simulink model "model_sysid_admittance"  (R2016b)
settings: Solver=FixedStepDiscrete  StartTime=0.0  StopTime=inf  FixedStep=sampleTime  RelTol=1e-3
PostLoadFcn:
  | % load model parameters
  | % pname = fileparts(get_param('model_base_bros','filename'));
  | % run([pname  '\parameters_base_model_bros.m']);
  | parameters_sysid_admittance;
  | 
  | % set requested state
  | set_param('model_sysid_admittance/Requested state','Value',num2str(0));
InitFcn:
  | % load model parameters
  | % pname = fileparts(get_param('model_base_bros','filename'));
  | % run([pname  '\parameters_base_model_bros.m']);
  | parameters_sysid_admittance;
  | 
  | % set requested state
  | set_param('model_sysid_admittance/Requested state','Value',num2str(0));
StartFcn:
  | parameters_sysid_admittance;
  | 
  | % set requested state
  | set_param('model_sysid_admittance/Requested state','Value',num2str(0));
values from neighbouring files (symbols this model uses):
  Ax = [0.00153392997769 0.00153392997769 0.00153392997769 0.00153392997769 0.00153392997769 0.00153392997769 0.00153392997769 0.00153392997769 0.00153392997769 0.00153392997769 0.00153392997769 0.00153392997769 ... (25 elements, 25x1)]    [data_inputsignal_admittance_100Hz.mat]
  Ay = [0.00153392997769 0.00153392997769 0.00153392997769 0.00153392997769 0.00153392997769 0.00153392997769 0.00153392997769 0.00153392997769 0.00153392997769 0.00153392997769 0.00153392997769 0.00153392997769 ... (25 elements, 25x1)]    [data_inputsignal_admittance_100Hz.mat]
  Lb = 0.07    [model_affc_parameters.m]    (also in parameters_sysid.m; parameters_sysid_admittance.m)
  Lf = 0.238    [model_affc_parameters.m]    (also in parameters_sysid.m; parameters_sysid_admittance.m)
  Lu = 0.153    [model_affc_parameters.m]    (also in parameters_sysid.m; parameters_sysid_admittance.m)
  nx = [5 7 11 13 17 23 29 37 47 61 79 103 ... (25 elements, 25x1)]    [data_inputsignal_admittance_100Hz.mat]
  ny = [3 8 10 14 19 24 31 41 53 67 83 107 ... (25 elements, 25x1)]    [data_inputsignal_admittance_100Hz.mat]
  phx = [1.20009664335 1.06282811403 1.3892882876 -0.190948998613 4.36135308948 3.55125265665 -1.29943418487 -0.0100316069113 1.01892216761 0.472716168264 1.16765179672 3.48382334533 ... (25 elements, 25x1)]    [data_inputsignal_admittance_100Hz.mat]
  phy = [4.61290873425 3.09865303555 -1.33576318949 -0.454866147562 0.315570179572 -1.54269258334 1.9231806523 3.28701306913 -0.551495079422 2.37779557242 1.0737629469 -1.42157877686 ... (25 elements, 25x1)]    [data_inputsignal_admittance_100Hz.mat]
  sampleTime = 0.001    [model_affc_parameters.m]    (also in parameters_sysid.m; parameters_sysid_admittance.m)
  Tm = 12    [data_inputsignal.mat]    (also in data_inputsignal_100Hz.mat; data_inputsignal_100Hz_n40.mat; data_inputsignal_150Hz_n50.mat; data_inputsignal_50Hz.mat)
undefined symbols (not defined in the file or in its folder): BROS3
libraries: simulink x14, LibraryFM x7, VariousBlocksLibrary x6, simulink_extras x1
(part 1 of 2)
settings Model: SimulationMode=external  Creator=niekbeckers  LastModifiedBy=Labuser
settings DataIOCC: LimitDataPoints=on  SaveFormat=Array
settings OptimizationCC: BlockReduction=off  BooleanDataType=off  LocalBlockOutputs=off  LifeSpan=inf
settings DebuggingCC: SaveWithParameterizedLinksMsg=none  UnderspecifiedInitializationDetection=Classic  MergeDetectMultiDrivingBlocksExec=none  SignalResolutionControl=TryResolveAllWithWarning  SFUnexpectedBacktrackingDiag=warning  SFNoUnconditionalDefaultTransitionDiag=warning  SFExecutionAtInitializationDiag=none
settings HardwareCC: ProdBitPerPointer=32  ProdBitPerSizeT=32  ProdBitPerPtrDiffT=32  ProdLargestAtomicFloat=None  ProdIntDivRoundTo=Undefined  ProdEndianess=Unspecified  ProdWordSize=32  ProdHWDeviceType=32-bit Generic  TargetBitPerPointer=64  TargetBitPerSizeT=64  TargetBitPerPtrDiffT=64  TargetLongLongMode=on  TargetIntDivRoundTo=Zero  TargetEndianess=LittleEndian  TargetWordSize=64  TargetHWDeviceType=MATLAB Host  ProdEqTarget=off
settings ModelReferenceCC: PropagateSignalLabelsOutOfModel=off
settings RTWCC: SystemTargetFile=TwinCAT.tlc  GenCodeOnly=on  MakeCommand=make_tct  TemplateMakefile=tct_msbuild.tmf  Description=TwinCAT Target  GenerateReport=on  TargetLang=C++
settings STFCustomTargetCC: CompOptLevelCompliant=on  GeneratePreprocessorConditionals=Disable all  MATLABClassNameForMDSCustomization=Simulink.SoftwareTarget.TargetSpecificTriggerConfigurationBase  SystemTargetFile=TwinCAT.tlc
settings ConfigComp: CovMetricSettings=dw  CovHtmlReporting=on  CovSaveCumulativeToWorkspaceVar=on  CovSaveSingleToWorkspaceVar=on  CovExternalEMLEnable=off  CovSFcnEnable=off

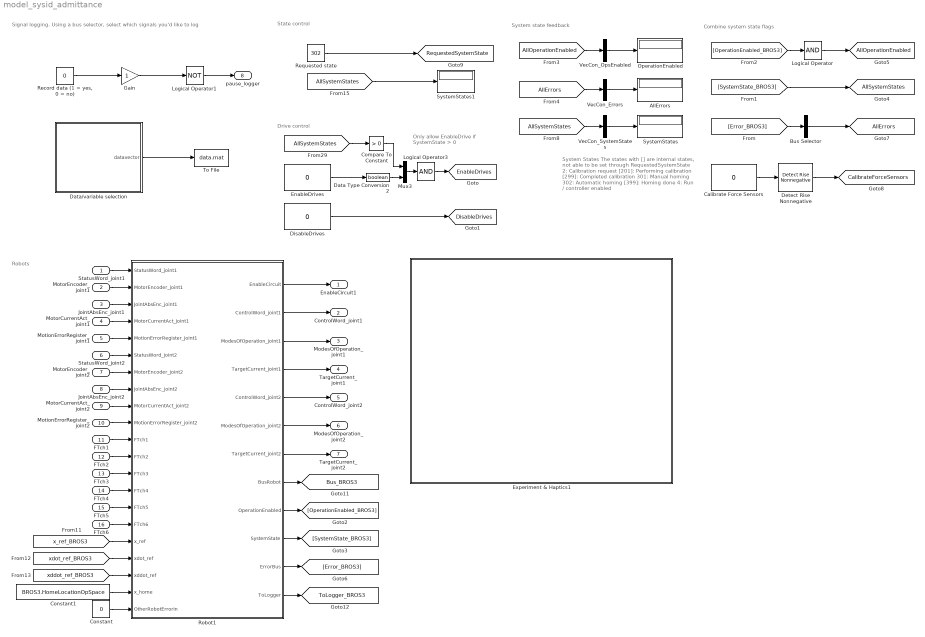
== system model_sysid_admittance ==
  note: Drive control
  note: System state feedback
  note: Only allow EnableDrive
      | if SystemState > 0
  note: Signal logging.
      | Using a bus selector, select which signals you'd like to log
  note: System States
      | The states with [] are internal states, not able to be set through RequestedSystemState
      | 2: Calibration request
      | [201]: Performing calibration
      | [299]: Completed calibration
      | 301: Manual homing
      | 302: Automatic homing
      | [399]: Homing done
      | 4: Run / controller enabled
  note: State control
  note: Combine system state flags
  note: Robots
  StatusWord_joint1 : Inport  OutDataTypeStr=uint16  PortDimensions=1
  MotorEncoder_joint1 : Inport  Port=2  OutDataTypeStr=int32  PortDimensions=1
  JointAbsEnc_joint1 : Inport  Port=3  OutDataTypeStr=int32  PortDimensions=1
  MotorCurrentAct_joint1 : Inport  Port=4  OutDataTypeStr=int16  PortDimensions=1
  MotionErrorRegister_joint1 : Inport  Port=5  OutDataTypeStr=uint16  PortDimensions=1
  StatusWord_joint2 : Inport  Port=6  OutDataTypeStr=uint16  PortDimensions=1
  MotorEncoder_joint2 : Inport  Port=7  OutDataTypeStr=int32  PortDimensions=1
  JointAbsEnc_joint2 : Inport  Port=8  OutDataTypeStr=int32  PortDimensions=1
  MotorCurrentAct_joint2 : Inport  Port=9  OutDataTypeStr=int16  PortDimensions=1
  MotionErrorRegister_joint2 : Inport  Port=10  OutDataTypeStr=uint16  PortDimensions=1
  FTch1 : Inport  Port=11  OutDataTypeStr=single  PortDimensions=1
  FTch2 : Inport  Port=12  OutDataTypeStr=single  PortDimensions=1
  FTch3 : Inport  Port=13  OutDataTypeStr=single  PortDimensions=1
  FTch4 : Inport  Port=14  OutDataTypeStr=single  PortDimensions=1
  FTch5 : Inport  Port=15  OutDataTypeStr=single  PortDimensions=1
  FTch6 : Inport  Port=16  OutDataTypeStr=single  PortDimensions=1
  AllErrors : Display
  Bus Selector : BusSelector  OutputSignals=ErrorCodeLatched  OutputAsBus=on
  Calibrate Force Sensors : Constant  Value=0
      settings: OpenFcn=set_param(gcb,'Value','1');tname = ['toggletimer_' gcb];delete(timerfind('name',tname));t = timer('timerfcn', ['set_param(''',gcb,''',''Value'',''0'')'],'executionmode','singleshot','startdelay',1,'name',tname);start(t);
      mask Display: fprintf('PushToTrigger\n%s',get_param(gcb,'value'))
  Compare To Constant : simulink/Logic and Bit Operations/Compare To Constant  relop=>  const=0  OutDataTypeStr=boolean
  Constant : Constant  Value=0
  Constant1 : Constant  Value=BROS3.HomeLocationOpSpace
  Data Type Conversion2 : DataTypeConversion  OutDataTypeStr=boolean
  Data/variable selection : Subsystem
  Detect Rise Nonnegative : simulink/Logic and Bit Operations/Detect Rise Nonnegative  vinit=0  OutDataTypeStr=boolean
  DisableDrives : Constant  Value=0
      settings: OpenFcn=set_param(gcb,'Value','1');tname = ['toggletimer_' gcb];delete(timerfind('name',tname));t = timer('timerfcn', ['set_param(''',gcb,''',''Value'',''0'')'],'executionmode','singleshot','startdelay',1,'name',tname);start(t);
      mask Display: fprintf('PushToTrigger\n%s',get_param(gcb,'value'))
  EnableDrives : Constant  Value=0
      settings: OpenFcn=set_param(gcb,'Value','1');tname = ['toggletimer_' gcb];delete(timerfind('name',tname));t = timer('timerfcn', ['set_param(''',gcb,''',''Value'',''0'')'],'executionmode','singleshot','startdelay',1,'name',tname);start(t);
      mask Display: fprintf('PushToTrigger\n%s',get_param(gcb,'value'))
  Experiment & Haptics1 : Subsystem
  Gain : Gain
  Logical Operator : Logic  Inputs=1  AllPortsSameDT=off  OutDataTypeStr=boolean
  Logical Operator1 : Logic  Operator=NOT  Inputs=1  AllPortsSameDT=off  OutDataTypeStr=boolean
  Logical Operator3 : Logic  Inputs=1  AllPortsSameDT=off  OutDataTypeStr=boolean
  Mux3 : Mux  Inputs=2
  OperationEnabled : Display
  "Record data (1 = yes, 0 = no)" : Constant  Value=0  OutDataTypeStr=boolean
  Requested state : Constant  Value=302
  Robot1 : Subsystem  mask{RobotStruct=BROS3}
      mask prompts: RobotStruct "Robot struct (data)"
  SystemStates : Display
  SystemStates1 : Display
  To File : ToFile  Filename=data.mat  MatrixName=data
  VecCon_Errors : Concatenate  NumInputs=1
  VecCon_OpsEnabled : Concatenate  NumInputs=1
  VecCon_SystemStates : Concatenate  NumInputs=1
  EnableCircuit1 : Outport  OutDataTypeStr=boolean  PortDimensions=1
  ControlWord_joint1 : Outport  Port=2  OutDataTypeStr=uint16  PortDimensions=1
  ModesOfOperation_joint1 : Outport  Port=3  OutDataTypeStr=int8  PortDimensions=1
  TargetCurrent_joint1 : Outport  Port=4  OutDataTypeStr=int16  PortDimensions=1
  ControlWord_joint2 : Outport  Port=5  OutDataTypeStr=uint16  PortDimensions=1
  ModesOfOperation_joint2 : Outport  Port=6  OutDataTypeStr=int8  PortDimensions=1
  TargetCurrent_joint2 : Outport  Port=7  OutDataTypeStr=int16  PortDimensions=1
  pause_logger : Outport  Port=8  OutDataTypeStr=boolean  PortDimensions=1
  tag scope: AllErrors=global, AllOperationEnabled=global, AllSystemStates=global, Bus_BROS3=global, CalibrateForceSensors=global, DisableDrives=global, EnableDrives=global, RequestedSystemState=global, ToLogger_BROS3=global
  wires:
  DisableDrives/1 -> [DisableDrives]
  Robot1/9(OperationEnabled) -> [OperationEnabled_BROS3]
  [AllOperationEnabled] -> VecCon_OpsEnabled/1
  Robot1/10(SystemState) -> [SystemState_BROS3]
  [SystemState_BROS3] -> [AllSystemStates]
  Logical Operator/1 -> [AllOperationEnabled]
  [OperationEnabled_BROS3] -> Logical Operator/1
  [Error_BROS3] -> Bus Selector/1
  [AllErrors] -> VecCon_Errors/1
  [x_ref_BROS3] -> Robot1/17(x_ref)
  [xdot_ref_BROS3] -> Robot1/18(xdot_ref)
  [xddot_ref_BROS3] -> Robot1/19(xddot_ref)
  Requested state/1 -> [RequestedSystemState]
  Robot1/8(BusRobot) -> [Bus_BROS3]
  StatusWord_joint1/1 -> Robot1/1(StatusWord_joint1)
  MotorEncoder_joint1/1 -> Robot1/2(MotorEncoder_joint1)
  JointAbsEnc_joint1/1 -> Robot1/3(JointAbsEnc_joint1)
  MotorCurrentAct_joint1/1 -> Robot1/4(MotorCurrentAct_joint1)
  StatusWord_joint2/1 -> Robot1/6(StatusWord_joint2)
  MotorEncoder_joint2/1 -> Robot1/7(MotorEncoder_joint2)
  JointAbsEnc_joint2/1 -> Robot1/8(JointAbsEnc_joint2)
  MotorCurrentAct_joint2/1 -> Robot1/9(MotorCurrentAct_joint2)
  FTch1/1 -> Robot1/11(FTch1)
  FTch2/1 -> Robot1/12(FTch2)
  FTch3/1 -> Robot1/13(FTch3)
  FTch4/1 -> Robot1/14(FTch4)
  FTch5/1 -> Robot1/15(FTch5)
  FTch6/1 -> Robot1/16(FTch6)
  Robot1/2(ControlWord_joint1) -> ControlWord_joint1/1
  Robot1/3(ModesOfOperation_joint1) -> ModesOfOperation_joint1/1
  Robot1/4(TargetCurrent_joint1) -> TargetCurrent_joint1/1
  Robot1/7(TargetCurrent_joint2) -> TargetCurrent_joint2/1
  Robot1/6(ModesOfOperation_joint2) -> ModesOfOperation_joint2/1
  Robot1/5(ControlWord_joint2) -> ControlWord_joint2/1
  [AllSystemStates] -> SystemStates1/1
  Logical Operator1/1 -> pause_logger/1
  Bus Selector/1 -> [AllErrors]
  Robot1/1(EnableCircuit) -> EnableCircuit1/1
  VecCon_Errors/1 -> AllErrors/1
  [AllSystemStates] -> VecCon_SystemStates/1
  VecCon_SystemStates/1 -> SystemStates/1
  VecCon_OpsEnabled/1 -> OperationEnabled/1
  [AllSystemStates] -> Compare To Constant/1
  Logical Operator3/1 -> [EnableDrives]
  EnableDrives/1 -> Data Type Conversion2/1
  Compare To Constant/1 -> Mux3/1
  Mux3/1 -> Logical Operator3/1
  Data Type Conversion2/1 -> Mux3/2
  Constant1/1 -> Robot1/20(x_home)
  Data/variable selection/1(datavector) -> To File/1
  Constant/1 -> Robot1/21(OtherRobotErrorIn)
  Calibrate Force Sensors/1 -> Detect Rise Nonnegative/1
  Detect Rise Nonnegative/1 -> [CalibrateForceSensors]
  Robot1/12(ToLogger) -> [ToLogger_BROS3]
  Robot1/11(ErrorBus) -> [Error_BROS3]
  MotionErrorRegister_joint1/1 -> Robot1/5(MotionErrorRegister_joint1)
  MotionErrorRegister_joint2/1 -> Robot1/10(MotionErrorRegister_joint2)
  "Record data (1 = yes, 0 = no)"/1 -> Gain/1
  Gain/1 -> Logical Operator1/1

== system model_sysid_admittance/Data//variable selection ==
  Bus to Vector : BusToVector
  BusSelectorLoggerBROS1 : BusSelector  OutputSignals=SystemState,qJointSpace.q_AbsEnc,qJointSpace.qdot_AbsEnc,qJointSpace.q_IncEnc,qJointSpace.qdot_IncEnc,xOpSpace.x_AbsEnc,xOpSpace.xdot_AbsEnc,xOpSpace.x,xOpSpace.xdot,Controller_ToLogger.x_ref,Controller_ToLogger.xdot_ref,Controller_ToLogger.xddot_ref,qJointSpace.JointTorque_Nm,BusFTSensor.ForcesOpSpace  OutputAsBus=on
  Mux5 : Mux  Inputs=3
  datavector : Outport
  wires:
  BusSelectorLoggerBROS1/1 -> Bus to Vector/1
  [ToLogger_BROS3] -> BusSelectorLoggerBROS1/1
  [AllErrors] -> Mux5/2
  Bus to Vector/1 -> Mux5/1
  Mux5/1 -> datavector/1
  [ExpData] -> Mux5/3

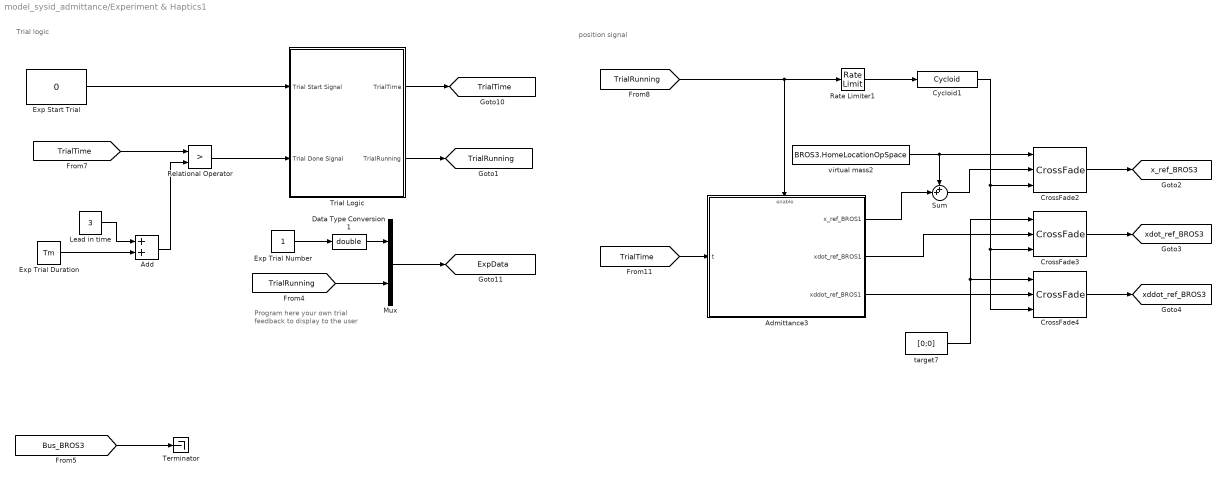
== system model_sysid_admittance/Experiment & Haptics1 ==
  note: Program here your own trial
      | feedback to display to the user
  note: Trial logic
  note: position signal
  Add : Sum
  Admittance3 : Subsystem
  CrossFade2 : VariousBlocksLibrary/Various/CrossFade
  CrossFade3 : VariousBlocksLibrary/Various/CrossFade
  CrossFade4 : VariousBlocksLibrary/Various/CrossFade
  Cycloid1 : VariousBlocksLibrary/Various/Cycloid
  Data Type Conversion1 : DataTypeConversion  OutDataTypeStr=double
  Exp Start Trial : Constant  Value=0
      settings: OpenFcn=set_param(gcb,'Value','1');tname = ['toggletimer_' gcb];delete(timerfind('name',tname));t = timer('timerfcn', ['set_param(''',gcb,''',''Value'',''0'')'],'executionmode','singleshot','startdelay',1,'name',tname);start(t);
      mask Display: fprintf('PushToTrigger\n%s',get_param(gcb,'value'))
  Exp Trial Duration : Constant  Value=Tm  OutDataTypeStr=double
  Exp Trial Number : Constant  OutDataTypeStr=int32
  Lead in time : Constant  Value=3  OutDataTypeStr=double
  Mux : Mux  Inputs=2
  Rate Limiter1 : RateLimiter  RisingSlewLimit=1/3.0  FallingSlewLimit=-1/3.0  SampleTimeMode=inherited
  Relational Operator : RelationalOperator  Operator=>  OutDataTypeStr=boolean  RndMeth=Simplest
  Sum : Sum  Inputs=++|
  Terminator : Terminator
  Trial Logic : Subsystem
  target7 : Constant  Value=[0;0]
  virtual mass2 : Constant  Value=BROS3.HomeLocationOpSpace
  tag scope: ExpData=global, TrialRunning=global, TrialTime=global, x_ref_BROS3=global, xddot_ref_BROS3=global, xdot_ref_BROS3=global
  wires:
  Mux/1 -> [ExpData]
  Exp Trial Number/1 -> Data Type Conversion1/1
  [TrialRunning] -> Mux/2
  Data Type Conversion1/1 -> Mux/1
  Exp Trial Duration/1 -> Add/2
  Exp Start Trial/1 -> Trial Logic/1(Trial Start Signal)
  Trial Logic/1(TrialTime) -> [TrialTime]
  Trial Logic/2(TrialRunning) -> [TrialRunning]
  Relational Operator/1 -> Trial Logic/2(Trial Done Signal)
  CrossFade2/1 -> [x_ref_BROS3]
  CrossFade3/1 -> [xdot_ref_BROS3]
  CrossFade4/1 -> [xddot_ref_BROS3]
  Add/1 -> Relational Operator/2
  Lead in time/1 -> Add/1
  [TrialTime] -> Relational Operator/1
  [TrialRunning] -> Rate Limiter1/1, Admittance3/Enable
  Cycloid1/1 -> CrossFade3/3, CrossFade4/3, CrossFade2/3
  Rate Limiter1/1 -> Cycloid1/1
  virtual mass2/1 -> CrossFade2/1, Sum/1
  target7/1 -> CrossFade3/1, CrossFade4/1
  Admittance3/2(xdot_ref_BROS1) -> CrossFade3/2
  Admittance3/3(xddot_ref_BROS1) -> CrossFade4/2
  [TrialTime] -> Admittance3/1(t)
  Admittance3/1(x_ref_BROS1) -> Sum/2
  Sum/1 -> CrossFade2/2
  [Bus_BROS3] -> Terminator/1

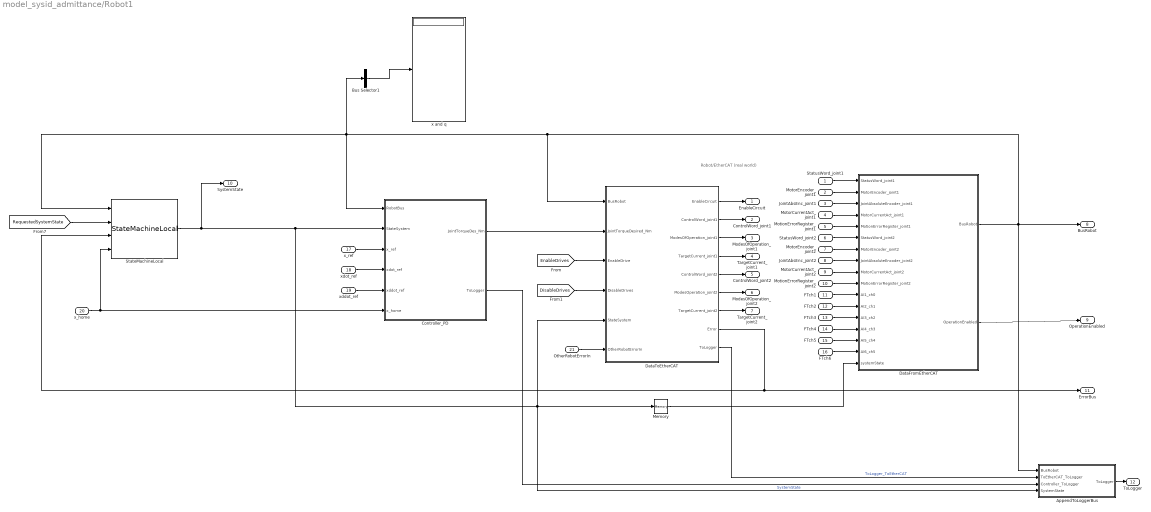
== system model_sysid_admittance/Robot1 ==
  note: Robot/EtherCAT (real world)
  StatusWord_joint1 : Inport
  MotorEncoder_joint1 : Inport  Port=2
  JointAbsEnc_joint1 : Inport  Port=3
  MotorCurrentAct_joint1 : Inport  Port=4
  MotionErrorRegister_joint1 : Inport  Port=5  OutDataTypeStr=uint16
  StatusWord_joint2 : Inport  Port=6
  MotorEncoder_joint2 : Inport  Port=7
  JointAbsEnc_joint2 : Inport  Port=8
  MotorCurrentAct_joint2 : Inport  Port=9
  MotionErrorRegister_joint2 : Inport  Port=10  OutDataTypeStr=uint16
  FTch1 : Inport  Port=11
  FTch2 : Inport  Port=12
  FTch3 : Inport  Port=13
  FTch4 : Inport  Port=14
  FTch5 : Inport  Port=15
  FTch6 : Inport  Port=16
  x_ref : Inport  Port=17
  xdot_ref : Inport  Port=18
  xddot_ref : Inport  Port=19
  x_home : Inport  Port=20
  OtherRobotErrorIn : Inport  Port=21
  AppendToLoggerBus : Subsystem
  Bus Selector1 : BusSelector  OutputSignals=qJointSpace.q_AbsEnc,qJointSpace.qdot_AbsEnc,xOpSpace.x,BusActuators.BusActuator1.JointPosition_AbsEnc_rad,BusActuators.BusActuator2.JointPosition_AbsEnc_rad,qJointSpace.q_IncEnc,qJointSpace.qdot_IncEnc  OutputAsBus=on
  Controller_PD : Subsystem
  DataFromEtherCAT : Subsystem
  DataToEtherCAT : Subsystem
  Memory : Memory
  StateMachineLocal : LibraryFM/StateMachineLocal
  x and q : Display
  EnableCircuit : Outport
  ControlWord_joint1 : Outport  Port=2
  ModesOfOperation_joint1 : Outport  Port=3
  TargetCurrent_joint1 : Outport  Port=4
  ControlWord_joint2 : Outport  Port=5
  ModesOfOperation_joint2 : Outport  Port=6
  TargetCurrent_joint2 : Outport  Port=7
  BusRobot : Outport  Port=8
  OperationEnabled : Outport  Port=9
  SystemState : Outport  Port=10
  ErrorBus : Outport  Port=11
  ToLogger : Outport  Port=12
  wires:
  xddot_ref/1 -> Controller_PD/5(xddot_ref)
  xdot_ref/1 -> Controller_PD/4(xdot_ref)
  x_ref/1 -> Controller_PD/3(x_ref)
  DataToEtherCAT/7(TargetCurrent_joint2) -> TargetCurrent_joint2/1
  FTch2/1 -> DataFromEtherCAT/12(AI2_ch1)
  MotorCurrentAct_joint1/1 -> DataFromEtherCAT/4(MotorCurrentAct_joint1)
  MotorEncoder_joint2/1 -> DataFromEtherCAT/7(MotorEncoder_joint2)
  JointAbsEnc_joint1/1 -> DataFromEtherCAT/3(JointAbsoluteEncoder_joint1)
  DataToEtherCAT/3(ModesOfOperation_joint1) -> ModesOfOperation_joint1/1
  DataToEtherCAT/1(EnableCircuit) -> EnableCircuit/1
  FTch1/1 -> DataFromEtherCAT/11(AI1_ch0)
  StateMachineLocal/1 -> Controller_PD/2(StateSystem), DataToEtherCAT/5(StateSystem), Memory/1, AppendToLoggerBus/4(SystemState), SystemState/1  "SystemState"
  DataToEtherCAT/2(ControlWord_joint1) -> ControlWord_joint1/1
  DataToEtherCAT/8(Error) -> StateMachineLocal/3, ErrorBus/1
  DataFromEtherCAT/1(BusRobot) -> AppendToLoggerBus/1(BusRobot), Controller_PD/1(RobotBus), Bus Selector1/1, StateMachineLocal/1, DataToEtherCAT/1(BusRobot), BusRobot/1
  [RequestedSystemState] -> StateMachineLocal/2
  Controller_PD/1(JointTorqueDes_Nm) -> DataToEtherCAT/2(JointTorqueDesired_Nm)
  [DisableDrives] -> DataToEtherCAT/4(DisableDrives)
  [EnableDrives] -> DataToEtherCAT/3(EnableDrive)
  MotorCurrentAct_joint2/1 -> DataFromEtherCAT/9(MotorCurrentAct_joint2)
  DataToEtherCAT/4(TargetCurrent_joint1) -> TargetCurrent_joint1/1
  FTch5/1 -> DataFromEtherCAT/15(AI5_ch4)
  JointAbsEnc_joint2/1 -> DataFromEtherCAT/8("JointAbsoluteEncoder_joint2 ")
  MotorEncoder_joint1/1 -> DataFromEtherCAT/2(MotorEncoder_joint1)
  DataToEtherCAT/5(ControlWord_joint2) -> ControlWord_joint2/1
  DataToEtherCAT/6(ModesOperation_joint2) -> ModesOfOperation_joint2/1
  StatusWord_joint1/1 -> DataFromEtherCAT/1(StatusWord_joint1)
  StatusWord_joint2/1 -> DataFromEtherCAT/6(StatusWord_joint2)
  FTch6/1 -> DataFromEtherCAT/16(AI6_ch5)
  FTch4/1 -> DataFromEtherCAT/14(AI4_ch3)
  FTch3/1 -> DataFromEtherCAT/13(AI3_ch2)
  DataFromEtherCAT/2(OperationEnabled) -> OperationEnabled/1
  Bus Selector1/1 -> x and q/1
  Controller_PD/2(ToLogger) -> AppendToLoggerBus/3(Controller_ToLogger)
  DataToEtherCAT/9(ToLogger) -> AppendToLoggerBus/2(ToEtherCAT_ToLogger)  "ToLogger_ToEtherCAT"
  AppendToLoggerBus/1(ToLogger) -> ToLogger/1
  Memory/1 -> DataFromEtherCAT/17(systemState)
  OtherRobotErrorIn/1 -> DataToEtherCAT/6(OtherRobotErrorIn)
  x_home/1 -> StateMachineLocal/4, Controller_PD/6(x_home)
  MotionErrorRegister_joint1/1 -> DataFromEtherCAT/5(MotionErrorRegister_joint1)
  MotionErrorRegister_joint2/1 -> DataFromEtherCAT/10(MotionErrorRegister_joint2)

== system model_sysid_admittance/Experiment & Haptics1/Admittance3 ==
  t : Inport
  Enable : EnablePort  StatesWhenEnabling=reset
  Constant3 : Constant  Value=0.5
  MATLAB Function : MATLAB Function  TreatAsAtomicUnit=on
  Product : Product
  Product1 : Product
  Product2 : Product
  x_ref_BROS1 : Outport
  xdot_ref_BROS1 : Outport  Port=2
  xddot_ref_BROS1 : Outport  Port=3
  wires:
  Product/1 -> x_ref_BROS1/1
  MATLAB Function/1(p) -> Product/2
  t/1 -> MATLAB Function/1(t)
  Product1/1 -> xdot_ref_BROS1/1
  Product2/1 -> xddot_ref_BROS1/1
  MATLAB Function/2(v) -> Product1/2
  MATLAB Function/3(a) -> Product2/2
  Constant3/1 -> Product2/1, Product1/1, Product/1

== system model_sysid_admittance/Experiment & Haptics1/Trial Logic ==
  Trial Start Signal : Inport
  Trial Done Signal : Inport  Port=2
  CheckTrialIsRunning : simulink_extras/Flip Flops/S-R Flip-Flop  initial_condition=0
  Data Type Conversion : DataTypeConversion  OutDataTypeStr=double
  Detect Rise Positive : simulink/Logic and Bit Operations/Detect Rise Positive  vinit=0  OutDataTypeStr=boolean
  Detect Rise Positive1 : simulink/Logic and Bit Operations/Detect Rise Positive  vinit=0  OutDataTypeStr=boolean
  Logical Operator : Logic  AllPortsSameDT=off  OutDataTypeStr=boolean
  Memory : Memory
  StopWatch : Subsystem
  Terminator4 : Terminator
  TrialTime : Outport
  TrialRunning : Outport  Port=2
  wires:
  CheckTrialIsRunning/1 -> Memory/1, Data Type Conversion/1
  Memory/1 -> StopWatch/Enable, Logical Operator/1
  Trial Start Signal/1 -> Detect Rise Positive/1
  Detect Rise Positive1/1 -> CheckTrialIsRunning/2
  Detect Rise Positive/1 -> CheckTrialIsRunning/1
  StopWatch/1(trialTime) -> TrialTime/1
  CheckTrialIsRunning/2 -> Terminator4/1
  Data Type Conversion/1 -> TrialRunning/1
  Trial Done Signal/1 -> Logical Operator/2
  Logical Operator/1 -> Detect Rise Positive1/1

== system model_sysid_admittance/Robot1/AppendToLoggerBus ==
  BusRobot : Inport
  ToEtherCAT_ToLogger : Inport  Port=2
  Controller_ToLogger : Inport  Port=3
  SystemState : Inport  Port=4
  Bus Creator : BusCreator  Inputs=8
  Bus Selector : BusSelector  OutputSignals=xOpSpace,qJointSpace,BusFTSensor,BusActuators
  Bus Selector1 : BusSelector  OutputSignals=ToEtherCAT_ToLogger_Actuator1,ToEtherCAT_ToLogger_Actuator2
  ToLogger : Outport
  wires:
  Bus Creator/1 -> ToLogger/1  "LoggerBus"
  Bus Selector/4 -> Bus Creator/4  "<BusActuators>"
  Bus Selector/1 -> Bus Creator/1  "<xOpSpace>"
  Bus Selector/3 -> Bus Creator/3  "<BusFTSensor>"
  Bus Selector/2 -> Bus Creator/2  "<qJointSpace>"
  BusRobot/1 -> Bus Selector/1
  ToEtherCAT_ToLogger/1 -> Bus Selector1/1
  Bus Selector1/1 -> Bus Creator/5  "<ToEtherCAT_ToLogger_Actuator1>"
  Bus Selector1/2 -> Bus Creator/6  "<ToEtherCAT_ToLogger_Actuator2>"
  Controller_ToLogger/1 -> Bus Creator/7
  SystemState/1 -> Bus Creator/8  "SystemState"

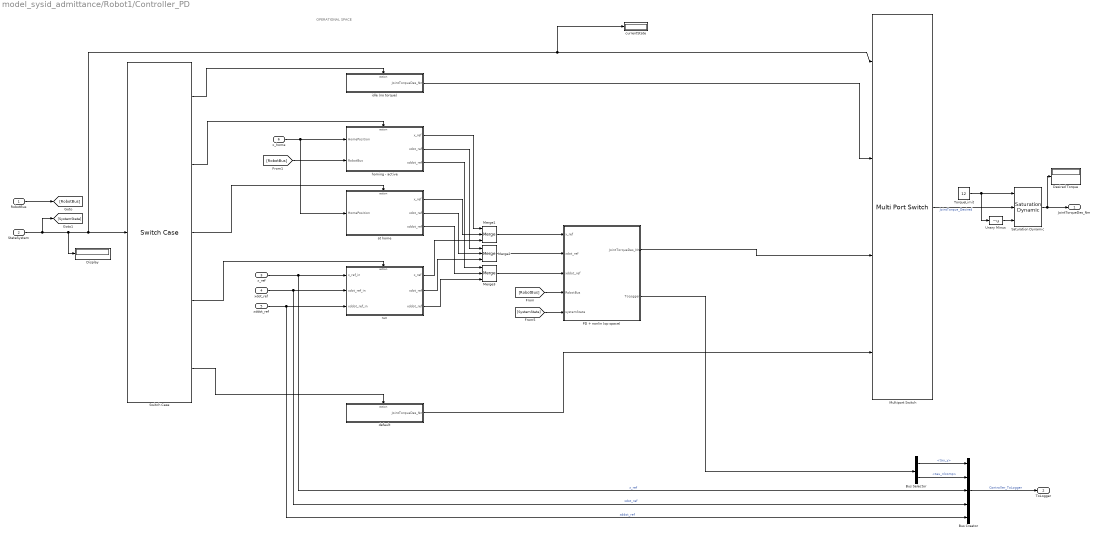
== system model_sysid_admittance/Robot1/Controller_PD ==
  note: OPERATIONAL SPACE
  RobotBus : Inport
  StateSystem : Inport  Port=2
  x_ref : Inport  Port=3
  xdot_ref : Inport  Port=4
  xddot_ref : Inport  Port=5
  x_home : Inport  Port=6
  Bus Creator : BusCreator  Inputs=5
  Bus Selector : BusSelector  OutputSignals=tau_y,tau_nlcomp
  Desired Torque : Display
  Display : Display
  Merge1 : Merge  Inputs=3  InitialOutput=[0;0]
  Merge2 : Merge  Inputs=3  InitialOutput=[0;0]
  Merge3 : Merge  Inputs=3  InitialOutput=[0;0]
  Multiport Switch : MultiPortSwitch  DataPortOrder=Specify indices  Inputs=4  DataPortIndices={[0,1,2,201,299,301],[302,399,4]}  DataPortForDefault=Additional data port
  PD + nonlin (op space) : Subsystem
  Saturation Dynamic : simulink/Discontinuities/Saturation Dynamic  OutMin=[]  OutMax=[]  OutDataTypeStr=Inherit: Same as second input  OutDataType=fixdt(1, 16)  OutScaling=2^-10  DoSatur=off
  Switch Case : SwitchCase  CaseConditions={[0,1,2,201,299,301],302, 399,[4]}
  TorqueLimit : Constant  Value=12
  Unary Minus : UnaryMinus
  at home : Subsystem
  currentState : Display
  default : Subsystem  TreatAsAtomicUnit=on
  homing - active : Subsystem
  idle (no torque) : Subsystem  TreatAsAtomicUnit=on
  run : Subsystem
  JointTorqueDes_Nm : Outport
  ToLogger : Outport  Port=2
  wires:
  [SystemState] -> PD + nonlin (op space)/5(systemState)
  xddot_ref/1 -> Bus Creator/5, run/3(xddot_ref_in)  "xddot_ref"
  xdot_ref/1 -> Bus Creator/4, run/2(xdot_ref_in)  "xdot_ref"
  x_ref/1 -> Bus Creator/3, run/1(x_ref_in)  "x_ref"
  [RobotBus] -> PD + nonlin (op space)/4(RobotBus)
  RobotBus/1 -> [RobotBus]
  Merge3/1 -> PD + nonlin (op space)/3(xddot_ref)
  Merge2/1 -> PD + nonlin (op space)/2(xdot_ref)
  Merge1/1 -> PD + nonlin (op space)/1(x_ref)
  idle (no torque)/1(JointTorqueDes_Nm) -> Multiport Switch/2
  Switch Case/2 -> homing - active/Action
  Switch Case/1 -> idle (no torque)/Action
  default/1(JointTorqueDes_Nm) -> Multiport Switch/4
  Switch Case/5 -> default/Action
  Saturation Dynamic/1 -> Desired Torque/1, JointTorqueDes_Nm/1
  Switch Case/3 -> at home/Action
  homing - active/1(x_ref) -> Merge1/1
  run/1(x_ref) -> Merge1/3
  StateSystem/1 -> Display/1, Multiport Switch/1, currentState/1, Switch Case/1, [SystemState]
  run/2(xdot_ref) -> Merge2/3
  run/3(xddot_ref) -> Merge3/3
  homing - active/2(xdot_ref) -> Merge2/1
  homing - active/3(xddot_ref) -> Merge3/1
  Multiport Switch/1 -> Saturation Dynamic/2  "JointTorque_Desired"
  PD + nonlin (op space)/2(ToLogger) -> Bus Selector/1
  x_home/1 -> at home/1(HomePosition), homing - active/1(HomePosition)
  Bus Creator/1 -> ToLogger/1  "Controller_ToLogger"
  Bus Selector/1 -> Bus Creator/1  "<tau_y>"
  Bus Selector/2 -> Bus Creator/2  "<tau_nlcomp>"
  TorqueLimit/1 -> Unary Minus/1, Saturation Dynamic/1
  Unary Minus/1 -> Saturation Dynamic/3
  [RobotBus] -> homing - active/2(RobotBus)
  at home/1(x_ref) -> Merge1/2
  at home/2(xdot_ref) -> Merge2/2
  at home/3(xddot_ref) -> Merge3/2
  Switch Case/4 -> run/Action
  PD + nonlin (op space)/1(JointTorqueDes_Nm) -> Multiport Switch/3

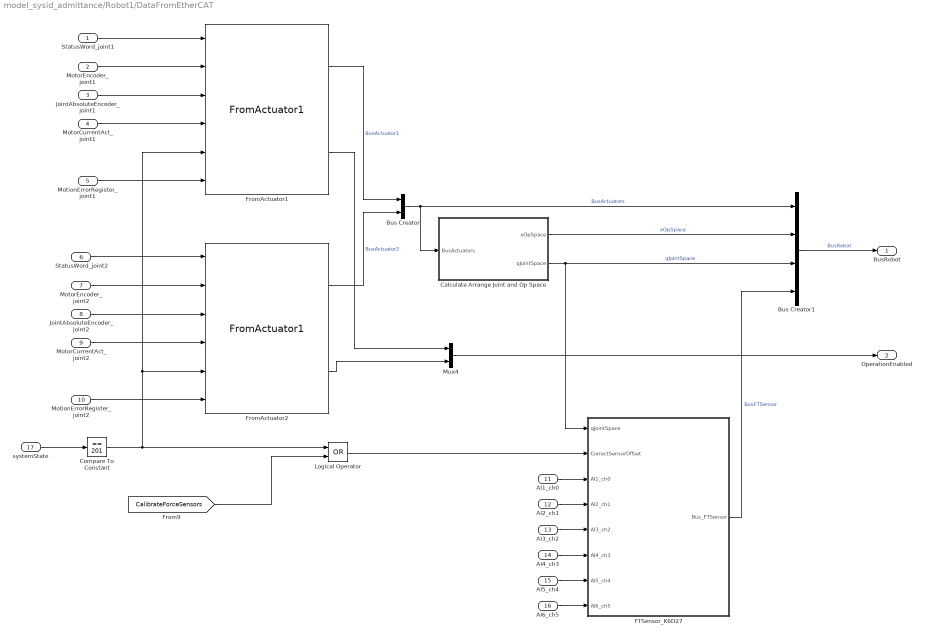
== system model_sysid_admittance/Robot1/DataFromEtherCAT ==
  StatusWord_joint1 : Inport
  MotorEncoder_joint1 : Inport  Port=2
  JointAbsoluteEncoder_joint1 : Inport  Port=3
  MotorCurrentAct_joint1 : Inport  Port=4
  MotionErrorRegister_joint1 : Inport  Port=5  OutDataTypeStr=uint16
  StatusWord_joint2 : Inport  Port=6
  MotorEncoder_joint2 : Inport  Port=7
  "JointAbsoluteEncoder_joint2 " : Inport  Port=8
  MotorCurrentAct_joint2 : Inport  Port=9
  MotionErrorRegister_joint2 : Inport  Port=10  OutDataTypeStr=uint16
  AI1_ch0 : Inport  Port=11
  AI2_ch1 : Inport  Port=12
  AI3_ch2 : Inport  Port=13
  AI4_ch3 : Inport  Port=14
  AI5_ch4 : Inport  Port=15
  AI6_ch5 : Inport  Port=16
  systemState : Inport  Port=17
  Bus Creator : BusCreator  Inputs=2
  Bus Creator1 : BusCreator  Inputs=4
  Calculate Arrange Joint and Op Space : Subsystem
  Compare To Constant : simulink/Logic and Bit Operations/Compare To Constant  relop===  const=201  OutDataTypeStr=boolean
  FTSensor_K6D27 : Subsystem  mask{FTSensorStruct=RobotStruct.FTSensor}
      mask prompts: FTSensorStruct "Struct for force torque sensor"
  FromActuator1 : LibraryFM/FromActuator1  ActuatorStruct=RobotStruct.Actuator1
  FromActuator2 : LibraryFM/FromActuator1  ActuatorStruct=RobotStruct.Actuator2
  Logical Operator : Logic  Operator=OR  AllPortsSameDT=off  OutDataTypeStr=boolean
  Mux4 : Mux  Inputs=2
  BusRobot : Outport
  OperationEnabled : Outport  Port=2
  wires:
  FTSensor_K6D27/1(Bus_FTSensor) -> Bus Creator1/4  "BusFTSensor"
  FromActuator1/1 -> Bus Creator/1  "BusActuator1"
  FromActuator2/1 -> Bus Creator/2  "BusActuator2"
  FromActuator1/2 -> Mux4/1
  Mux4/1 -> OperationEnabled/1
  FromActuator2/2 -> Mux4/2
  MotorEncoder_joint1/1 -> FromActuator1/2
  StatusWord_joint1/1 -> FromActuator1/1
  JointAbsoluteEncoder_joint1/1 -> FromActuator1/3
  MotorCurrentAct_joint1/1 -> FromActuator1/4
  MotorEncoder_joint2/1 -> FromActuator2/2
  StatusWord_joint2/1 -> FromActuator2/1
  "JointAbsoluteEncoder_joint2 "/1 -> FromActuator2/3
  MotorCurrentAct_joint2/1 -> FromActuator2/4
  Bus Creator/1 -> Calculate Arrange Joint and Op Space/1(BusActuators), Bus Creator1/1  "BusActuators"
  Bus Creator1/1 -> BusRobot/1  "BusRobot"
  Calculate Arrange Joint and Op Space/2(qJointSpace) -> FTSensor_K6D27/1(qJointSpace), Bus Creator1/3  "qJointSpace"
  systemState/1 -> Compare To Constant/1
  AI1_ch0/1 -> FTSensor_K6D27/3(AI1_ch0)
  AI2_ch1/1 -> FTSensor_K6D27/4(AI2_ch1)
  AI3_ch2/1 -> FTSensor_K6D27/5(AI3_ch2)
  AI4_ch3/1 -> FTSensor_K6D27/6(AI4_ch3)
  AI5_ch4/1 -> FTSensor_K6D27/7(AI5_ch4)
  AI6_ch5/1 -> FTSensor_K6D27/8(AI6_ch5)
  Compare To Constant/1 -> Logical Operator/1, FromActuator1/5, FromActuator2/5
  Calculate Arrange Joint and Op Space/1(xOpSpace) -> Bus Creator1/2  "xOpSpace"
  [CalibrateForceSensors] -> Logical Operator/2
  Logical Operator/1 -> FTSensor_K6D27/2(CorrectSensorOffset)
  MotionErrorRegister_joint1/1 -> FromActuator1/6
  MotionErrorRegister_joint2/1 -> FromActuator2/6

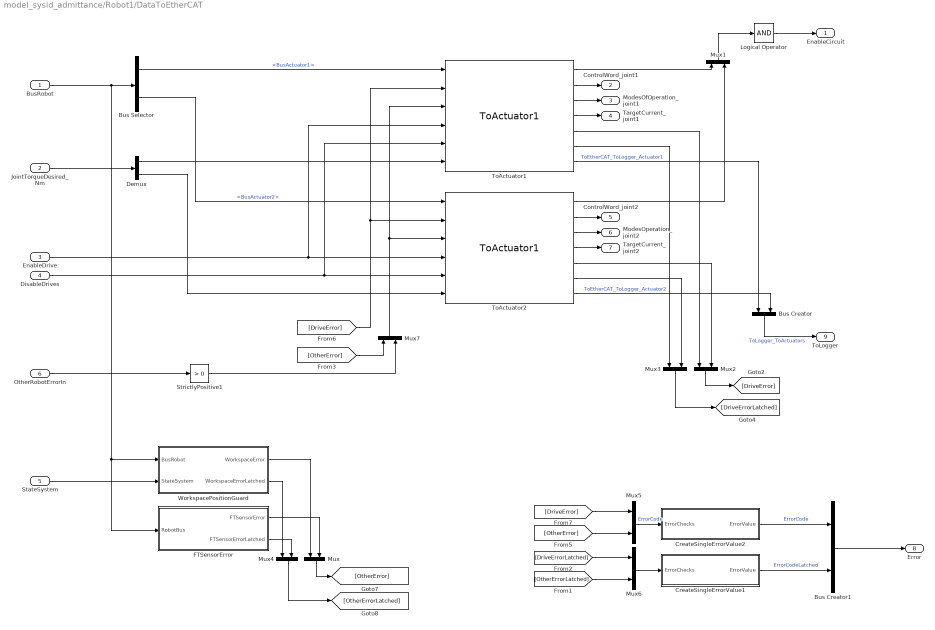
== system model_sysid_admittance/Robot1/DataToEtherCAT ==
  BusRobot : Inport
  JointTorqueDesired_Nm : Inport  Port=2
  EnableDrive : Inport  Port=3
  DisableDrives : Inport  Port=4
  StateSystem : Inport  Port=5
  OtherRobotErrorIn : Inport  Port=6
  Bus Creator : BusCreator  Inputs=2
  Bus Creator1 : BusCreator  Inputs=2
  Bus Selector : BusSelector  OutputSignals=BusActuators.BusActuator1,BusActuators.BusActuator2
  CreateSingleErrorValue1 : Subsystem
  CreateSingleErrorValue2 : Subsystem
  Demux : Demux  Outputs=2
  FTSensorError : Subsystem
  Logical Operator : Logic  Inputs=1  AllPortsSameDT=off  OutDataTypeStr=boolean
  Mux{,1..7} (8 alike) : Mux  Inputs=2
  StrictlyPositive1 : simulink/Logic and Bit Operations/Compare To Zero  relop=>  OutDataTypeStr=boolean
  ToActuator1 : LibraryFM/ToActuator1  ActuatorStruct=RobotStruct.Actuator1
  ToActuator2 : LibraryFM/ToActuator1  ActuatorStruct=RobotStruct.Actuator2
  WorkspacePositionGuard : Subsystem
  EnableCircuit : Outport  OutDataTypeStr=boolean
  ControlWord_joint1 : Outport  Port=2  OutDataTypeStr=uint16
  ModesOfOperation_joint1 : Outport  Port=3  OutDataTypeStr=int8
  TargetCurrent_joint1 : Outport  Port=4  OutDataTypeStr=int16
  ControlWord_joint2 : Outport  Port=5  OutDataTypeStr=uint16
  ModesOperation_joint2 : Outport  Port=6  OutDataTypeStr=int8
  TargetCurrent_joint2 : Outport  Port=7  OutDataTypeStr=int16
  Error : Outport  Port=8
  ToLogger : Outport  Port=9
  wires:
  Bus Creator/1 -> ToLogger/1  "ToLogger_ToActuators"
  ToActuator2/7 -> Bus Creator/2  "ToEtherCAT_ToLogger_Actuator2"
  ToActuator1/7 -> Bus Creator/1  "ToEtherCAT_ToLogger_Actuator1"
  ToActuator1/5 -> Mux2/1
  ToActuator2/5 -> Mux2/2
  Mux2/1 -> [DriveError]
  ToActuator1/6 -> Mux3/1
  ToActuator2/6 -> Mux3/2
  [DriveError] -> ToActuator1/2, ToActuator2/2
  Mux1/1 -> Logical Operator/1
  ToActuator1/1 -> Mux1/1
  ToActuator2/1 -> Mux1/2
  ToActuator1/2 -> ControlWord_joint1/1
  ToActuator1/3 -> ModesOfOperation_joint1/1
  ToActuator2/2 -> ControlWord_joint2/1
  ToActuator1/4 -> TargetCurrent_joint1/1
  ToActuator2/4 -> TargetCurrent_joint2/1
  ToActuator2/3 -> ModesOperation_joint2/1
  Logical Operator/1 -> EnableCircuit/1
  Demux/2 -> ToActuator2/6
  JointTorqueDesired_Nm/1 -> Demux/1
  Demux/1 -> ToActuator1/6
  BusRobot/1 -> WorkspacePositionGuard/1(BusRobot), FTSensorError/1(RobotBus), Bus Selector/1
  Bus Selector/2 -> ToActuator2/1  "<BusActuator2>"
  Bus Selector/1 -> ToActuator1/1  "<BusActuator1>"
  DisableDrives/1 -> ToActuator1/5, ToActuator2/5
  EnableDrive/1 -> ToActuator1/4, ToActuator2/4
  Mux3/1 -> [DriveErrorLatched]
  StateSystem/1 -> WorkspacePositionGuard/2(StateSystem)
  FTSensorError/1(FTSensorError) -> Mux/2
  FTSensorError/2(FTSensorErrorLatched) -> Mux4/2
  WorkspacePositionGuard/1(WorkspaceError) -> Mux/1
  WorkspacePositionGuard/2(WorkspaceErrorLatched) -> Mux4/1
  Mux/1 -> [OtherError]
  Mux4/1 -> [OtherErrorLatched]
  [DriveError] -> Mux5/1
  [OtherError] -> Mux5/2
  CreateSingleErrorValue1/1(ErrorValue) -> Bus Creator1/2  "ErrorCodeLatched"
  [DriveErrorLatched] -> Mux6/1
  [OtherErrorLatched] -> Mux6/2
  Mux6/1 -> CreateSingleErrorValue1/1(ErrorChecks)
  Mux5/1 -> CreateSingleErrorValue2/1(ErrorChecks)  "ErrorCode"
  Bus Creator1/1 -> Error/1
  CreateSingleErrorValue2/1(ErrorValue) -> Bus Creator1/1  "ErrorCode"
  [OtherError] -> Mux7/1
  Mux7/1 -> ToActuator2/3, ToActuator1/3
  OtherRobotErrorIn/1 -> StrictlyPositive1/1
  StrictlyPositive1/1 -> Mux7/2

== system model_sysid_admittance/Experiment & Haptics1/Trial Logic/StopWatch ==
  Enable : EnablePort  StatesWhenEnabling=reset
  Counter Free-Running : simulink/Sources/Counter Free-Running  NumBits=32  tsamp=-1
  Data Type Conversion : DataTypeConversion  OutDataTypeStr=double
  sample time : Gain  Gain=sampleTime
  trialTime : Outport
  wires:
  sample time/1 -> trialTime/1
  Data Type Conversion/1 -> sample time/1
  Counter Free-Running/1 -> Data Type Conversion/1

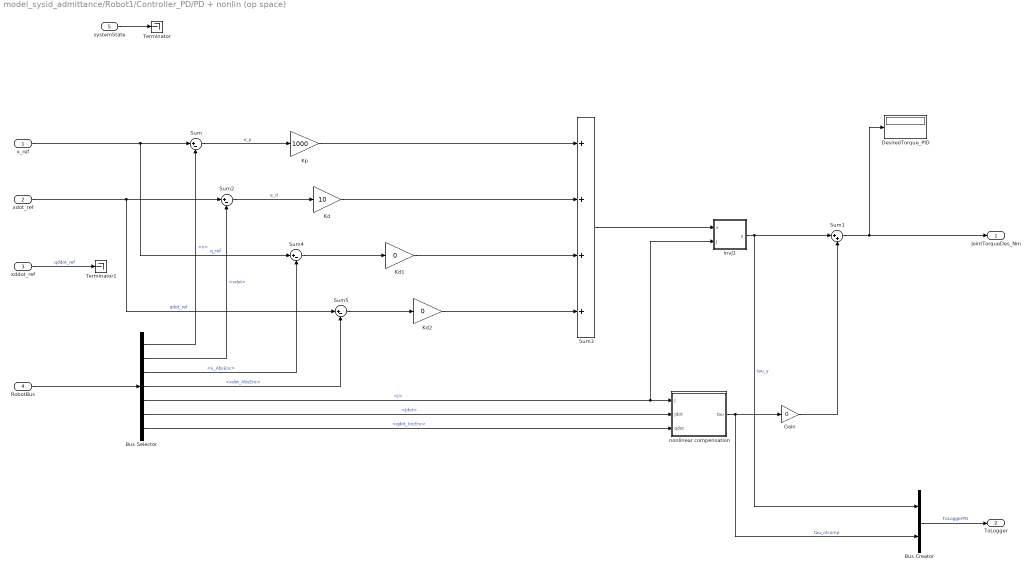
== system model_sysid_admittance/Robot1/Controller_PD/PD + nonlin (op space) ==
  x_ref : Inport
  xdot_ref : Inport  Port=2
  xddot_ref : Inport  Port=3
  RobotBus : Inport  Port=4
  systemState : Inport  Port=5
  Bus Creator : BusCreator  Inputs=2
  Bus Selector : BusSelector  OutputSignals=xOpSpace.x,xOpSpace.xdot,xOpSpace.x_AbsEnc,xOpSpace.xdot_AbsEnc,xOpSpace.J,xOpSpace.Jdot,qJointSpace.qdot_IncEnc
  DesiredTorque_PID : Display
  Gain : Gain  Gain=0
  Kd : Gain  Gain=10
  Kd1 : Gain  Gain=0
  Kd2 : Gain  Gain=0
  Kp : Gain  Gain=1000
  Sum{,2,4..5} (4 alike) : Sum  Inputs=|+-
  Sum1 : Sum  Inputs=|++
  Sum3 : Sum  Inputs=++++
  Terminator : Terminator
  Terminator1 : Terminator
  invJ1 : MATLAB Function  TreatAsAtomicUnit=on
  nonlinear compensation : MATLAB Function  TreatAsAtomicUnit=on
  JointTorqueDes_Nm : Outport
  ToLogger : Outport  Port=2
  wires:
  nonlinear compensation/1(tau) -> Gain/1, Bus Creator/2  "tau_nlcomp"
  invJ1/1(y) -> Sum1/1, Bus Creator/1  "tau_y"
  Bus Selector/1 -> Sum/2  "<x>"
  x_ref/1 -> Sum/1, Sum4/1  "q_ref"
  Sum/1 -> Kp/1  "e_p"
  xdot_ref/1 -> Sum5/1, Sum2/1  "qdot_ref"
  Sum2/1 -> Kd/1  "e_d"
  Sum1/1 -> JointTorqueDes_Nm/1, DesiredTorque_PID/1
  systemState/1 -> Terminator/1
  Bus Creator/1 -> ToLogger/1  "ToLoggerPD"
  Gain/1 -> Sum1/2
  Bus Selector/2 -> Sum2/2  "<xdot>"
  Bus Selector/6 -> nonlinear compensation/2(Jdot)  "<Jdot>"
  Bus Selector/5 -> nonlinear compensation/1(J), invJ1/2(J)  "<J>"
  RobotBus/1 -> Bus Selector/1
  Sum4/1 -> Kd1/1
  Sum5/1 -> Kd2/1
  xddot_ref/1 -> Terminator1/1  "qddot_ref"
  Bus Selector/3 -> Sum4/2  "<x_AbsEnc>"
  Bus Selector/4 -> Sum5/2  "<xdot_AbsEnc>"
  Kd/1 -> Sum3/2
  Kp/1 -> Sum3/1
  Sum3/1 -> invJ1/1(x)
  Kd1/1 -> Sum3/3
  Kd2/1 -> Sum3/4
  Bus Selector/7 -> nonlinear compensation/3(qdot)  "<qdot_IncEnc>"

== system model_sysid_admittance/Robot1/Controller_PD/at home ==
  note: The velocity and acceleration references are set to [0;0] for stability.
  HomePosition : Inport
  Action Port : ActionPort  InitializeStates=reset  ActionType=case
  Constant : Constant
  Constant2 : Constant  Value=[0;0]
  Constant4 : Constant  Value=[0;0]
  HoldFirstSampleOnEnable : Subsystem
  x_ref : Outport  InitialOutput=[0;0]
  xdot_ref : Outport  Port=2  InitialOutput=[0;0]
  xddot_ref : Outport  Port=3  InitialOutput=[0;0]
  wires:
  Constant2/1 -> xdot_ref/1
  HoldFirstSampleOnEnable/1(x0) -> x_ref/1
  Constant4/1 -> xddot_ref/1
  Constant/1 -> HoldFirstSampleOnEnable/Enable
  HomePosition/1 -> HoldFirstSampleOnEnable/1(x)

== system model_sysid_admittance/Robot1/Controller_PD/default ==
  Action Port : ActionPort  InitializeStates=reset  ActionType=default
  Constant3 : Constant  Value=[0;0]
  JointTorqueDes_Nm : Outport  InitialOutput=[0;0]
  wires:
  Constant3/1 -> JointTorqueDes_Nm/1

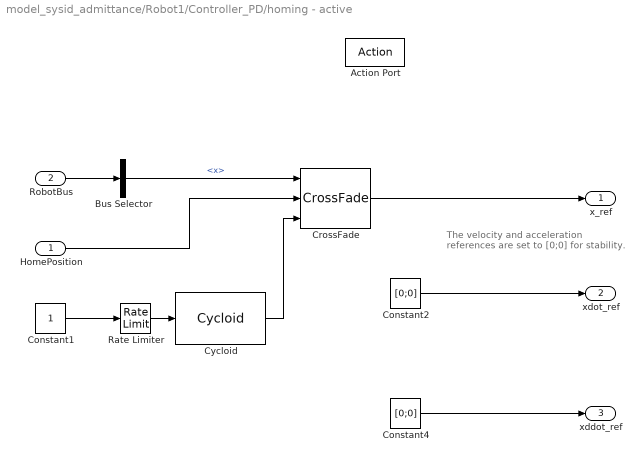
== system model_sysid_admittance/Robot1/Controller_PD/homing - active ==
  note: The velocity and acceleration references are set to [0;0] for stability.
  HomePosition : Inport
  RobotBus : Inport  Port=2
  Action Port : ActionPort  InitializeStates=reset  ActionType=case
  Bus Selector : BusSelector  OutputSignals=xOpSpace.x
  Constant1 : Constant
  Constant2 : Constant  Value=[0;0]
  Constant4 : Constant  Value=[0;0]
  CrossFade : VariousBlocksLibrary/Various/CrossFade
  Cycloid : VariousBlocksLibrary/Various/Cycloid
  Rate Limiter : RateLimiter  RisingSlewLimit=0.1  FallingSlewLimit=-0.2  SampleTimeMode=inherited
  x_ref : Outport  InitialOutput=[0;0]
  xdot_ref : Outport  Port=2  InitialOutput=[0;0]
  xddot_ref : Outport  Port=3  InitialOutput=[0;0]
  wires:
  Constant2/1 -> xdot_ref/1
  Bus Selector/1 -> CrossFade/1  "<x>"
  RobotBus/1 -> Bus Selector/1
  HomePosition/1 -> CrossFade/2
  Cycloid/1 -> CrossFade/3
  Rate Limiter/1 -> Cycloid/1
  Constant1/1 -> Rate Limiter/1
  CrossFade/1 -> x_ref/1
  Constant4/1 -> xddot_ref/1

== system model_sysid_admittance/Robot1/Controller_PD/idle (no torque) ==
  Action Port : ActionPort  InitializeStates=reset  ActionType=case
  Constant3 : Constant  Value=[0;0]
  JointTorqueDes_Nm : Outport  InitialOutput=[0;0]
  wires:
  Constant3/1 -> JointTorqueDes_Nm/1

== system model_sysid_admittance/Robot1/Controller_PD/run ==
  x_ref_in : Inport
  xdot_ref_in : Inport  Port=2
  xddot_ref_in : Inport  Port=3
  Action Port : ActionPort  InitializeStates=reset  ActionType=case
  x_ref : Outport  InitialOutput=[0;0]
  xdot_ref : Outport  Port=2  InitialOutput=[0;0]
  xddot_ref : Outport  Port=3  InitialOutput=[0;0]
  wires:
  xdot_ref_in/1 -> xdot_ref/1
  xddot_ref_in/1 -> xddot_ref/1
  x_ref_in/1 -> x_ref/1

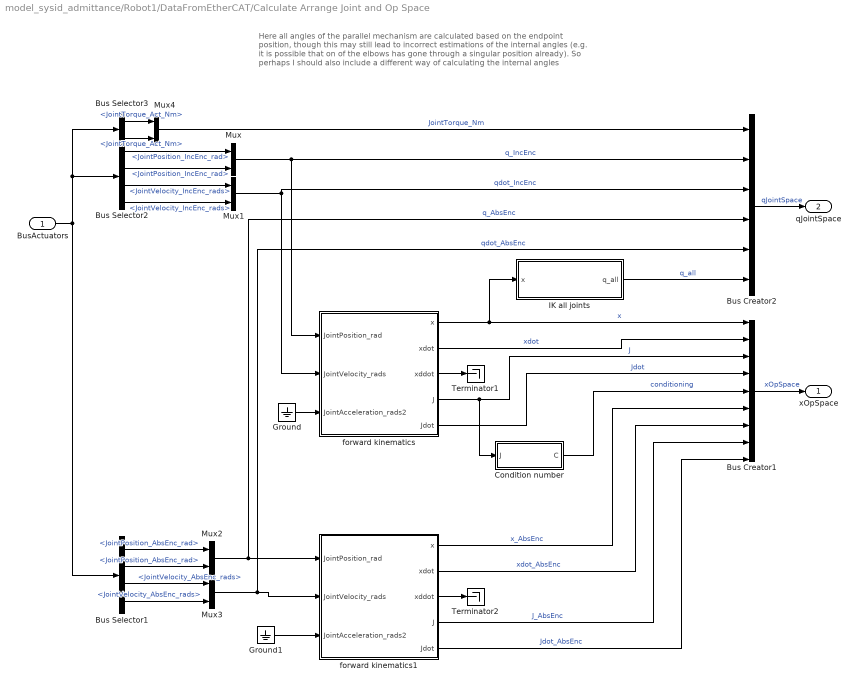
== system model_sysid_admittance/Robot1/DataFromEtherCAT/Calculate Arrange Joint and Op Space ==
  note: Here all angles of the parallel mechanism are calculated
      | based on the endpoint position, though this may still lead to incorrect
      | estimations of the internal angles (e.g. it is possible that on of the elbows
      | has gone through a singular position already). So perhaps I should also include
      | a different way of calculating the internal angles
  BusActuators : Inport
  Bus Creator1 : BusCreator  Inputs=9
  Bus Creator2 : BusCreator  Inputs=6
  Bus Selector1 : BusSelector  OutputSignals=BusActuator1.JointPosition_AbsEnc_rad,BusActuator2.JointPosition_AbsEnc_rad,BusActuator1.JointVelocity_AbsEnc_rads,BusActuator2.JointVelocity_AbsEnc_rads
  Bus Selector2 : BusSelector  OutputSignals=BusActuator1.JointPosition_IncEnc_rad,BusActuator2.JointPosition_IncEnc_rad,BusActuator1.JointVelocity_IncEnc_rads,BusActuator2.JointVelocity_IncEnc_rads
  Bus Selector3 : BusSelector  OutputSignals=BusActuator1.JointTorque_Act_Nm,BusActuator2.JointTorque_Act_Nm
  Condition number : MATLAB Function  TreatAsAtomicUnit=on
  Ground : Ground
  Ground1 : Ground
  IK all joints : MATLAB Function  TreatAsAtomicUnit=on
  Mux{,1..4} (5 alike) : Mux  Inputs=2
  Terminator1 : Terminator
  Terminator2 : Terminator
  forward kinematics : Subsystem
  forward kinematics1 : Subsystem
  xOpSpace : Outport
  qJointSpace : Outport  Port=2
  wires:
  forward kinematics/5(Jdot) -> Bus Creator1/4  "Jdot"
  forward kinematics/3(xddot) -> Terminator1/1
  forward kinematics/2(xdot) -> Bus Creator1/2  "xdot"
  forward kinematics/1(x) -> IK all joints/1(x), Bus Creator1/1  "x"
  Bus Creator1/1 -> xOpSpace/1  "xOpSpace"
  forward kinematics/4(J) -> Condition number/1(J), Bus Creator1/3  "J"
  Ground/1 -> forward kinematics/3(JointAcceleration_rads2)
  Bus Creator2/1 -> qJointSpace/1  "qJointSpace"
  BusActuators/1 -> Bus Selector1/1, Bus Selector3/1, Bus Selector2/1
  Bus Selector2/1 -> Mux/1  "<JointPosition_IncEnc_rad>"
  Bus Selector2/2 -> Mux/2  "<JointPosition_IncEnc_rad>"
  Bus Selector2/3 -> Mux1/1  "<JointVelocity_IncEnc_rads>"
  Bus Selector2/4 -> Mux1/2  "<JointVelocity_IncEnc_rads>"
  Mux1/1 -> Bus Creator2/3, forward kinematics/2(JointVelocity_rads)  "qdot_IncEnc"
  Mux/1 -> forward kinematics/1(JointPosition_rad), Bus Creator2/2  "q_IncEnc"
  IK all joints/1(q_all) -> Bus Creator2/6  "q_all"
  Condition number/1(C) -> Bus Creator1/5  "conditioning"
  Bus Selector1/4 -> Mux3/2  "<JointVelocity_AbsEnc_rads>"
  Bus Selector1/3 -> Mux3/1  "<JointVelocity_AbsEnc_rads>"
  Bus Selector1/2 -> Mux2/2  "<JointPosition_AbsEnc_rad>"
  Bus Selector1/1 -> Mux2/1  "<JointPosition_AbsEnc_rad>"
  forward kinematics1/3(xddot) -> Terminator2/1
  Ground1/1 -> forward kinematics1/3(JointAcceleration_rads2)
  Mux2/1 -> Bus Creator2/4, forward kinematics1/1(JointPosition_rad)  "q_AbsEnc"
  Mux3/1 -> Bus Creator2/5, forward kinematics1/2(JointVelocity_rads)  "qdot_AbsEnc"
  forward kinematics1/2(xdot) -> Bus Creator1/7  "xdot_AbsEnc"
  forward kinematics1/1(x) -> Bus Creator1/6  "x_AbsEnc"
  forward kinematics1/4(J) -> Bus Creator1/8  "J_AbsEnc"
  forward kinematics1/5(Jdot) -> Bus Creator1/9  "Jdot_AbsEnc"
  Bus Selector3/1 -> Mux4/1  "<JointTorque_Act_Nm>"
  Bus Selector3/2 -> Mux4/2  "<JointTorque_Act_Nm>"
  Mux4/1 -> Bus Creator2/1  "JointTorque_Nm"

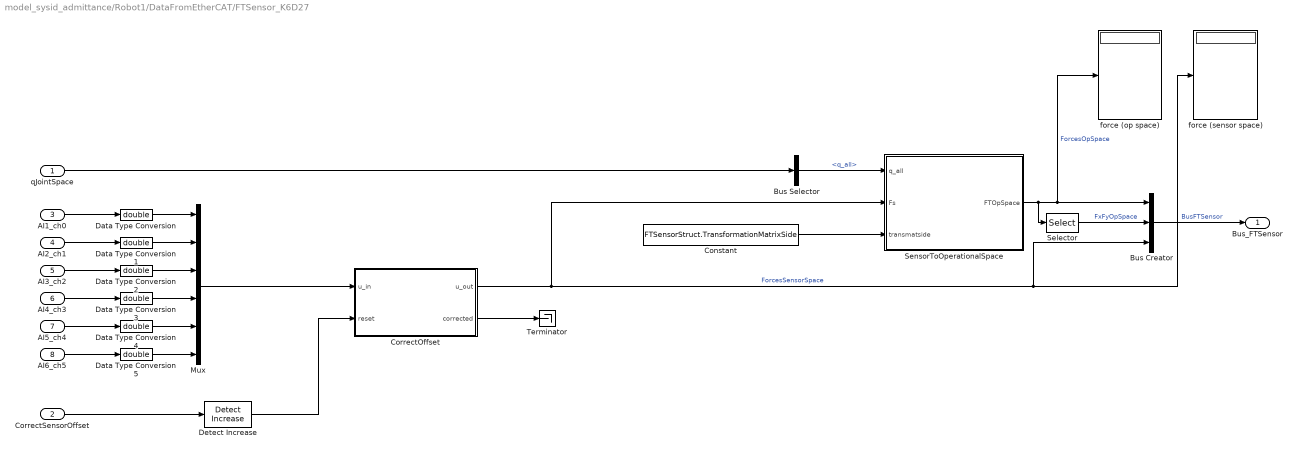
== system model_sysid_admittance/Robot1/DataFromEtherCAT/FTSensor_K6D27 ==
  qJointSpace : Inport
  CorrectSensorOffset : Inport  Port=2
  AI1_ch0 : Inport  Port=3
  AI2_ch1 : Inport  Port=4
  AI3_ch2 : Inport  Port=5
  AI4_ch3 : Inport  Port=6
  AI5_ch4 : Inport  Port=7
  AI6_ch5 : Inport  Port=8
  Bus Creator : BusCreator  Inputs=3
  Bus Selector : BusSelector  OutputSignals=q_all
  Constant : Constant  Value=FTSensorStruct.TransformationMatrixSide
  CorrectOffset : MATLAB Function  TreatAsAtomicUnit=on
  Data Type Conversion{,1..5} (6 alike) : DataTypeConversion  OutDataTypeStr=double
  Detect Increase : simulink/Logic and Bit Operations/Detect Increase  vinit=0.0  InputProcessing=Inherited  OutDataTypeStr=boolean
  Mux : Mux  Inputs=6
  Selector : Selector  InputPortWidth=6  IndexOptions=Index vector (dialog)  Indices=[1 2]  OutputSizes=1
  SensorToOperationalSpace : MATLAB Function  TreatAsAtomicUnit=on
  Terminator : Terminator
  force (op space) : Display
  force (sensor space) : Display
  Bus_FTSensor : Outport
  wires:
  Constant/1 -> SensorToOperationalSpace/3(transmatside)
  Bus Creator/1 -> Bus_FTSensor/1  "BusFTSensor"
  SensorToOperationalSpace/1(FTOpSpace) -> Selector/1, force (op space)/1, Bus Creator/1  "ForcesOpSpace"
  Data Type Conversion5/1 -> Mux/6
  Data Type Conversion4/1 -> Mux/5
  Data Type Conversion3/1 -> Mux/4
  Data Type Conversion2/1 -> Mux/3
  Data Type Conversion1/1 -> Mux/2
  Data Type Conversion/1 -> Mux/1
  CorrectOffset/1(u_out) -> SensorToOperationalSpace/2(Fs), Bus Creator/3, force (sensor space)/1  "ForcesSensorSpace"
  CorrectOffset/2(corrected) -> Terminator/1
  AI3_ch2/1 -> Data Type Conversion2/1
  AI4_ch3/1 -> Data Type Conversion3/1
  AI5_ch4/1 -> Data Type Conversion4/1
  AI6_ch5/1 -> Data Type Conversion5/1
  Detect Increase/1 -> CorrectOffset/2(reset)
  CorrectSensorOffset/1 -> Detect Increase/1
  Mux/1 -> CorrectOffset/1(u_in)
  AI1_ch0/1 -> Data Type Conversion/1
  AI2_ch1/1 -> Data Type Conversion1/1
  qJointSpace/1 -> Bus Selector/1
  Bus Selector/1 -> SensorToOperationalSpace/1(q_all)  "<q_all>"
  Selector/1 -> Bus Creator/2  "FxFyOpSpace"

== system model_sysid_admittance/Robot1/DataToEtherCAT/CreateSingleErrorValue1 ==
  ErrorChecks : Inport
  Data Type Conversion1 : DataTypeConversion  OutDataTypeStr=double
  ErrorToPower2 : MATLAB Function  TreatAsAtomicUnit=on
  ErrorValue : Outport
  wires:
  Data Type Conversion1/1 -> ErrorToPower2/1(u)
  ErrorChecks/1 -> Data Type Conversion1/1
  ErrorToPower2/1(e) -> ErrorValue/1

== system model_sysid_admittance/Robot1/DataToEtherCAT/CreateSingleErrorValue2 ==
  ErrorChecks : Inport
  Data Type Conversion1 : DataTypeConversion  OutDataTypeStr=double
  ErrorToPower2 : MATLAB Function  TreatAsAtomicUnit=on
  ErrorValue : Outport
  wires:
  Data Type Conversion1/1 -> ErrorToPower2/1(u)
  ErrorChecks/1 -> Data Type Conversion1/1
  ErrorToPower2/1(e) -> ErrorValue/1

== system model_sysid_admittance/Robot1/DataToEtherCAT/FTSensorError ==
  RobotBus : Inport
  AvoidAlgebraicLoop : Memory
  Bus Selector : BusSelector  OutputSignals=BusFTSensor.ForcesSensorSpace
  Constant : Constant  Value=RobotStruct.FTSensor.MaxAllowableForcesTorqueSensor
  Data Type Conversion1 : DataTypeConversion  OutDataTypeStr=boolean
  Detect Change : simulink/Logic and Bit Operations/Detect Change  vinit=0  InputProcessing=Inherited  OutDataTypeStr=boolean
  FTSensorLastError : Display
  LatchRising : LibraryFM/Utilities/LatchRising  ic=0
  MATLAB Function : MATLAB Function  TreatAsAtomicUnit=on
  ShowFTSensorErrorLatched : Display
  FTSensorError : Outport
  FTSensorErrorLatched : Outport  Port=2
  wires:
  Constant/1 -> MATLAB Function/2(MaxForcesTorques)
  MATLAB Function/1(e) -> Data Type Conversion1/1, FTSensorLastError/1
  LatchRising/1 -> ShowFTSensorErrorLatched/1, FTSensorErrorLatched/1
  AvoidAlgebraicLoop/1 -> Detect Change/1, LatchRising/1, FTSensorError/1
  Detect Change/1 -> LatchRising/Trigger
  RobotBus/1 -> Bus Selector/1
  Bus Selector/1 -> MATLAB Function/1(ForcesTorques)  "<ForcesSensorSpace>"
  Data Type Conversion1/1 -> AvoidAlgebraicLoop/1

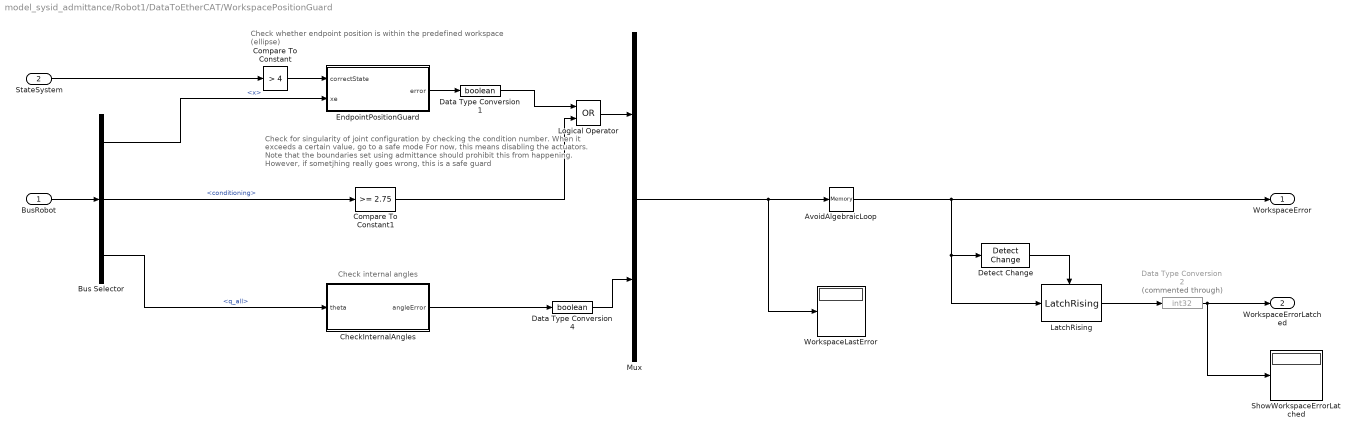
== system model_sysid_admittance/Robot1/DataToEtherCAT/WorkspacePositionGuard ==
  note: Check internal angles
  note: Check whether endpoint position is within the predefined workspace
      | (ellipse)
  note: Check for singularity of joint configuration by checking
      | the condition number. When it exceeds a certain value, go to a safe mode
      | For now, this means disabling the actuators.
      | Note that the boundaries set using admittance should prohibit this from happening.
      | However, if sometjhing really goes wrong, this is a safe guard
  BusRobot : Inport
  StateSystem : Inport  Port=2
  AvoidAlgebraicLoop : Memory
  Bus Selector : BusSelector  OutputSignals=xOpSpace.x,xOpSpace.conditioning,qJointSpace.q_all
  CheckInternalAngles : MATLAB Function  TreatAsAtomicUnit=on
  Compare To Constant : simulink/Logic and Bit Operations/Compare To Constant  relop=>  const=4  OutDataTypeStr=boolean
  Compare To Constant1 : simulink/Logic and Bit Operations/Compare To Constant  relop=>=  const=2.75  OutDataTypeStr=boolean
  Data Type Conversion1 : DataTypeConversion  OutDataTypeStr=boolean
  Data Type Conversion2 : DataTypeConversion  Commented=through  OutDataTypeStr=int32
  Data Type Conversion4 : DataTypeConversion  OutDataTypeStr=boolean
  Detect Change : simulink/Logic and Bit Operations/Detect Change  vinit=0  InputProcessing=Inherited  OutDataTypeStr=boolean
  EndpointPositionGuard : MATLAB Function  TreatAsAtomicUnit=on
  LatchRising : LibraryFM/Utilities/LatchRising  ic=0
  Logical Operator : Logic  Operator=OR  AllPortsSameDT=off  OutDataTypeStr=boolean
  Mux : Mux  Inputs=2
  ShowWorkspaceErrorLatched : Display
  WorkspaceLastError : Display
  WorkspaceError : Outport
  WorkspaceErrorLatched : Outport  Port=2
  wires:
  BusRobot/1 -> Bus Selector/1
  Bus Selector/1 -> EndpointPositionGuard/2(xe)  "<x>"
  LatchRising/1 -> Data Type Conversion2/1
  EndpointPositionGuard/1(error) -> Data Type Conversion1/1
  Mux/1 -> AvoidAlgebraicLoop/1, WorkspaceLastError/1
  Detect Change/1 -> LatchRising/Trigger
  AvoidAlgebraicLoop/1 -> WorkspaceError/1, Detect Change/1, LatchRising/1
  Compare To Constant/1 -> EndpointPositionGuard/1(correctState)
  Bus Selector/2 -> Compare To Constant1/1  "<conditioning>"
  StateSystem/1 -> Compare To Constant/1
  Data Type Conversion2/1 -> WorkspaceErrorLatched/1, ShowWorkspaceErrorLatched/1
  CheckInternalAngles/1(angleError) -> Data Type Conversion4/1
  Bus Selector/3 -> CheckInternalAngles/1(theta)  "<q_all>"
  Data Type Conversion4/1 -> Mux/2
  Logical Operator/1 -> Mux/1
  Data Type Conversion1/1 -> Logical Operator/1
  Compare To Constant1/1 -> Logical Operator/2

== system model_sysid_admittance/Robot1/Controller_PD/at home/HoldFirstSampleOnEnable ==
  note: These blocks hold the first sample of the input
      | when the block is enabled (through the action port)
  x : Inport
  Enable : EnablePort  StatesWhenEnabling=reset
  Counter Free-Running : simulink/Sources/Counter Free-Running  NumBits=32  tsamp=-1
  Memory1 : Memory
  Signal Conversion : SignalConversion  OverrideOpt=off
  Switch : Switch  Threshold=1
  x0 : Outport
  wires:
  x/1 -> Switch/3
  Counter Free-Running/1 -> Switch/2
  Memory1/1 -> Switch/1
  Switch/1 -> Signal Conversion/1, Memory1/1
  Signal Conversion/1 -> x0/1

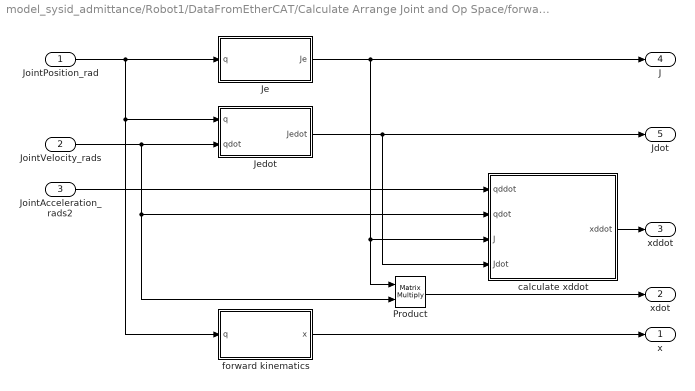
== system model_sysid_admittance/Robot1/DataFromEtherCAT/Calculate Arrange Joint and Op Space/forward kinematics ==
  JointPosition_rad : Inport  PortDimensions=[2 1]
  JointVelocity_rads : Inport  Port=2  PortDimensions=[2 1]
  JointAcceleration_rads2 : Inport  Port=3  PortDimensions=[2 1]
  Je : MATLAB Function  TreatAsAtomicUnit=on
  Jedot : MATLAB Function  TreatAsAtomicUnit=on
  Product : Product  Multiplication=Matrix(*)
  calculate xddot : MATLAB Function  TreatAsAtomicUnit=on
  forward kinematics : MATLAB Function  TreatAsAtomicUnit=on
  x : Outport
  xdot : Outport  Port=2
  xddot : Outport  Port=3
  J : Outport  Port=4
  Jdot : Outport  Port=5
  wires:
  JointPosition_rad/1 -> forward kinematics/1(q), Jedot/1(q), Je/1(q)
  Je/1(Je) -> calculate xddot/3(J), Product/1, J/1
  JointVelocity_rads/1 -> calculate xddot/2(qdot), Product/2, Jedot/2(qdot)
  Jedot/1(Jedot) -> calculate xddot/4(Jdot), Jdot/1
  Product/1 -> xdot/1
  forward kinematics/1(x) -> x/1
  calculate xddot/1(xddot) -> xddot/1
  JointAcceleration_rads2/1 -> calculate xddot/1(qddot)
